simulink model "BD_PAR_SS"  (Simulink 10.3)
settings: Solver=ode1  StartTime=0.0  StopTime=max(cyc_mph(:,1))  FixedStep=1  MaxStep=1  RelTol=1e-3  AbsTol=1e-3
undefined symbols (not defined in the file): acc_elec_eff, acc_elec_pwr, acc_mech_eff, amb_tmp, cs_charge_deplete_bool, cs_electric_decel_spd, cs_electric_launch_spd_hi, cs_electric_launch_spd_lo, cs_hi_soc, cs_lo_soc, cs_off_trq_frac, cyc_avg_time, cyc_cargo_mass, cyc_elevation_init, cyc_filter_bool, cyc_grade, cyc_mph, ess_module_num, ess_on, ess_voc, ex_calc, ex_cat_co_frac, ex_cat_ext_cp, ex_cat_ext_emisv, ex_cat_ext_init_tmp, ex_cat_ext_mass, ex_cat_ext_sarea, ex_cat_hc_frac, ex_cat_i2p_th_cond, ex_cat_i2x_emisv, ex_cat_i2x_th_cond, ex_cat_int_cp, ex_cat_int_init_tmp, ex_cat_int_mass, ex_cat_int_sarea, ex_cat_lim, ex_cat_m2i_th_cond, ex_cat_m2i_tmp, ex_cat_m2p_emisv, ex_cat_mon_cp, ex_cat_mon_init_tmp, ex_cat_mon_mass, ex_cat_mon_sarea, ex_cat_monf_sarea, ex_cat_moni_sarea, ex_cat_nox_frac, ex_cat_p2x_th_cond, ex_cat_pcm_ecp, ex_cat_pcm_mass, ex_cat_pcm_tmp, ex_cat_pipe_cp, ex_cat_pipe_emisv, ex_cat_pipe_init_tmp, ex_cat_pipe_mass, ex_cat_pipe_sarea, ex_cat_pm_frac, ex_cat_tmp_range, ex_gas_cp, ex_manif_cp, ex_manif_emisv ... (+73)
libraries: lib_controls x6, lib_vehicle x3, lib_accessory x2, lib_interactive x1, lib_energy_storage x1, lib_fuel_converter x1
(part 6 of 6)

== system BD_PAR_SS/exhaust sys <ex>/removal efficiencies/removal efficiencies ORNL/NOx_Eff ==
  vol_flow : Inport
  Ex_temp : Inport  Port=2
  HC_Inlet : Inport  Port=3
  NOx_Inlet : Inport  Port=4
  1 : Constant
  >eps : Saturate  UpperLimit=inf  LowerLimit=eps
  Gain : Gain  Gain=2.875  SaturateOnIntegerOverflow=on
  Gain1 : Gain  Gain=.01  SaturateOnIntegerOverflow=on
  HNR : Product  Inputs=*/  SaturateOnIntegerOverflow=on
  HNR^.5 : Math  Operator=sqrt  SaturateOnIntegerOverflow=on
  HNR^2 : Math  Operator=square  SaturateOnIntegerOverflow=on
  HNR^3 : Product  SaturateOnIntegerOverflow=on
  NOx_conv2 : Display
  SV^.5 : Math  Operator=sqrt  SaturateOnIntegerOverflow=on
  SV^2 : Math  Operator=square  SaturateOnIntegerOverflow=on
  SV^3 : Product  SaturateOnIntegerOverflow=on
  Saturation : Saturate  UpperLimit=1.0  LowerLimit=0.0
  Sum : Sum  Inputs=|+++++  SaturateOnIntegerOverflow=on
  Sum1 : Sum  Inputs=|++++  SaturateOnIntegerOverflow=on
  Sum2 : Sum  Inputs=|++++  SaturateOnIntegerOverflow=on
  Sum3 : Sum  Inputs=|+++  SaturateOnIntegerOverflow=on
  TR : Product  Inputs=*/  SaturateOnIntegerOverflow=on
  T^-.5 : Math  Operator=sqrt  SaturateOnIntegerOverflow=on
  T^-2 : Math  Operator=square  SaturateOnIntegerOverflow=on
  T^-3 : Product  SaturateOnIntegerOverflow=on
  b0 : Constant  Value=-1.2477959e2
  b1 : Gain  Gain=-6.671239E-4  SaturateOnIntegerOverflow=on
  b10 : Gain  Gain=-1.7874225E1  SaturateOnIntegerOverflow=on
  b11 : Gain  Gain=-2.0607707  SaturateOnIntegerOverflow=on
  b12 : Gain  Gain=1.3883777E-1  SaturateOnIntegerOverflow=on
  b13 : Gain  SaturateOnIntegerOverflow=on
  b2 : Gain  Gain=8.308073E-2  SaturateOnIntegerOverflow=on
  b3 : Gain  Gain=7.9852675E-9  SaturateOnIntegerOverflow=on
  b4 : Gain  Gain=-3.7023358E-14  SaturateOnIntegerOverflow=on
  b5 : Gain  Gain=-5.4929168E4  SaturateOnIntegerOverflow=on
  b6 : Gain  Gain=4.9229015e3  SaturateOnIntegerOverflow=on
  b7 : Gain  Gain=2.959987e6  SaturateOnIntegerOverflow=on
  b8 : Gain  Gain=-1.022441e8  SaturateOnIntegerOverflow=on
  b9 : Gain  Gain=1.3710201E1  SaturateOnIntegerOverflow=on
  NOx_eff : Outport
  wires:
  >eps/1 -> HNR/2
  NOx_Inlet/1 -> >eps/1
  Saturation/1 -> NOx_eff/1, NOx_conv2/1
  Ex_temp/1 -> TR/2
  HC_Inlet/1 -> HNR/1
  b13/1 -> SV^3/1, b1/1, SV^2/1, SV^.5/1
  Gain1/1 -> Saturation/1
  Sum3/1 -> Gain1/1
  Gain/1 -> HNR^2/1, HNR^3/2, b9/1, HNR^.5/1
  HNR/1 -> Gain/1
  Sum/1 -> Sum3/1
  Sum1/1 -> Sum3/2
  Sum2/1 -> Sum3/3
  b12/1 -> Sum2/4
  b11/1 -> Sum2/3
  b10/1 -> Sum2/2
  b9/1 -> Sum2/1
  HNR^.5/1 -> b10/1
  HNR^2/1 -> b11/1, HNR^3/1
  HNR^3/1 -> b12/1
  b8/1 -> Sum1/4
  b7/1 -> Sum1/3
  b6/1 -> Sum1/2
  b5/1 -> Sum1/1
  T^-.5/1 -> b6/1
  T^-2/1 -> b7/1, T^-3/1
  T^-3/1 -> b8/1
  TR/1 -> b5/1, T^-3/2, T^-2/1, T^-.5/1
  1/1 -> TR/1
  b3/1 -> Sum/5
  b4/1 -> Sum/4
  b1/1 -> Sum/3
  b2/1 -> Sum/2
  b0/1 -> Sum/1
  SV^.5/1 -> b2/1
  SV^2/1 -> b3/1, SV^3/2
  SV^3/1 -> b4/1
  vol_flow/1 -> b13/1

== system BD_PAR_SS/fuel converter  <fc>/engine speed estimator/no-lag Reset Integrator/dt ==
  Clock : Clock
  Memory1 : Memory  InitialCondition=-0.1
  Sum1 : Sum  Inputs=+-  InputSameDT=on  SaturateOnIntegerOverflow=on  OutDataTypeStr=Inherit: Same as first input
  out_1 : Outport  InitialOutput=0
  wires:
  Sum1/1 -> out_1/1
  Memory1/1 -> Sum1/2
  Clock/1 -> Memory1/1, Sum1/1

== system BD_PAR_SS/fuel converter  <fc>/engine torque/effect of inertia (Nm)/Block NOTES ==
  note: Torque required to accelerate the engine inertia is taken from the engine
      | acceleration, and is assumed to be no less than zero if the trace was missed
      | at all on the previous time step.
      |
      | The torque required to accelerate the engine's inertia is never assumed to
      | be more than the product of the engine's maximum torque and the engine's
      | contribution to the total vehicle inertia.

== system BD_PAR_SS/fuel converter  <fc>/engine torque/effect of inertia (Nm)/engine inertia as a function of total vehicle inertia (generous approximation) ==
  Product : Product  Inputs=*/  InputSameDT=on  RndMeth=Zero  SaturateOnIntegerOverflow=on  OutDataTypeStr=Inherit: Same as first input
  Sum : Sum  Inputs=++|  InputSameDT=on  SaturateOnIntegerOverflow=on  OutDataTypeStr=Inherit: Same as first input
  engine inertia as a fraction of total vehicle inertia  (generous approximation)--denomenator : Fcn  Expr=fc_inertia*(u*fd_ratio/wh_radius)^2
  engine inertia as a fraction of total vehicle inertia  (generous approximation)--numerator : Fcn  Expr=fc_inertia*(u*fd_ratio/wh_radius)^2
  veh mass calc : Subsystem
  Out1 : Outport
  wires:
  [gear_ratio] -> engine inertia as a fraction of total vehicle inertia  (generous approximation)--numerator/1, engine inertia as a fraction of total vehicle inertia  (generous approximation)--denomenator/1
  veh mass calc/1(Out1) -> Sum/1
  engine inertia as a fraction of total vehicle inertia  (generous approximation)--denomenator/1 -> Sum/2
  engine inertia as a fraction of total vehicle inertia  (generous approximation)--numerator/1 -> Product/1
  Sum/1 -> Product/2
  Product/1 -> Out1/1

== system BD_PAR_SS/gearbox <gb>/Pout/Pin, neglecting inertia/make division bombproof/Block NOTES ==
  note: this block added 10 July 2001 by mpo:
      | originally a -eps was added to the denominator by default.
      | However, cases were ecountered where Tin-Tineratia was equal to -eps causing
      | the denominator to be zero. This added checking is more rhobust

== system BD_PAR_SS/mechanical accessory loads <acc>/Mechanical Accessory Loads v2 <acc>/Accessory SDO/mechanical power logging ==
  In1 : Inport
  Gain : Gain  Gain=acc_mech_eff  SaturateOnIntegerOverflow=on  OutDataTypeStr=Inherit: Same as input  ParamDataTypeStr=Inherit: Same as input
  To Workspace6 : ToWorkspace  VariableName=acc_mech_pwr_in_a  SampleTime=-1
  To Workspace8 : ToWorkspace  VariableName=acc_mech_pwr_out_a  SampleTime=-1
  wires:
  Gain/1 -> To Workspace8/1
  In1/1 -> Gain/1, To Workspace6/1

== system BD_PAR_SS/mechanical accessory loads <acc>/Mechanical Accessory Loads v2 <acc>/backward model/mechanical accessories (Nm) ==
  w_APU : Inport
  Mechanical Accessories: Const Mech Var Elect : lib_accessory/Mechanical Accessories: Const Mech Var Elect  SystemSampleTime=-1  VariantActivationTime=update diagram  Latency=0  AutoFrameSizeCalculation=off
  T_acc : Outport
  P_mech_acc : Outport  Port=2
  probes : Outport  Port=3
  wires:
  w_APU/1 -> Mechanical Accessories: Const Mech Var Elect/1
  Mechanical Accessories: Const Mech Var Elect/1 -> T_acc/1
  Mechanical Accessories: Const Mech Var Elect/2 -> P_mech_acc/1
  Mechanical Accessories: Const Mech Var Elect/3 -> probes/1

== system BD_PAR_SS/motor/ controller <mc> par/effect of inertia (Nm)/motor inertia as a function of total vehicle inertia (generous approximation)/veh mass calc ==
  Constant : Constant  Value=veh_mass
  Sum : Sum  Inputs=|++  SaturateOnIntegerOverflow=on
  Out1 : Outport
  wires:
  Sum/1 -> Out1/1
  Constant/1 -> Sum/2
  [veh_cargo_mass] -> Sum/1

== system BD_PAR_SS/vehicle <veh>/record achieved force outputs/force req'd to accelerate (N)1/current veh mass ==
  Constant3 : Constant  Value=veh_mass
  Sum1 : Sum  Inputs=|++  SaturateOnIntegerOverflow=on
  Out1 : Outport
  wires:
  Constant3/1 -> Sum1/1
  [veh_cargo_mass] -> Sum1/2
  Sum1/1 -> Out1/1

== system BD_PAR_SS/vehicle <veh>/record achieved force outputs/force req'd to ascend (N)1/current veh mass ==
  Constant3 : Constant  Value=veh_mass
  Sum1 : Sum  Inputs=|++  SaturateOnIntegerOverflow=on
  Out1 : Outport
  wires:
  Constant3/1 -> Sum1/1
  [veh_cargo_mass] -> Sum1/2
  Sum1/1 -> Out1/1

== system BD_PAR_SS/<vc> par/pre-TX parallel gearbox control/shifting1/time since last shift/just shifted ==
  in_1 : Inport
  Memory : Memory  InitialCondition=1
  Relational Operator : RelationalOperator  Operator=~=  RndMeth=Nearest  InputSameDT=on
  out_1 : Outport  InitialOutput=0
  wires:
  in_1/1 -> Memory/1, Relational Operator/2
  Memory/1 -> Relational Operator/1
  Relational Operator/1 -> out_1/1

== system BD_PAR_SS/<vc> par/pre-TX parallel gearbox control/shifting1/time since last shift/timer ==
  trigger : Inport
  Constant : Constant
  Constant1 : Constant  Value=0
  Constant2 : Constant  Value=0
  Switch : Switch  Threshold=eps  SaturateOnIntegerOverflow=on  InputSameDT=on
  no-lag Reset Integrator : Subsystem  mask(No-lag Reset Integrator){initval=15}
      mask prompts: initval "Initial Value"
      mask help: No-lag Reset Integrator
      mask Help: Integrates first input using Euler technique.\nAt the time step that input 2 <> zero,\noutput is reset to input 3.
      mask Display: disp('1/s\nw/ reset\nno lag')
  time : Outport  InitialOutput=0
  wires:
  no-lag Reset Integrator/1(out_1) -> Switch/3
  Constant1/1 -> no-lag Reset Integrator/3(in_3)
  Constant/1 -> no-lag Reset Integrator/1(in_1)
  Constant2/1 -> Switch/1
  trigger/1 -> no-lag Reset Integrator/2(in_2), Switch/2
  Switch/1 -> time/1

== system BD_PAR_SS/fuel converter  <fc>/engine torque/effect of inertia (Nm)/engine inertia as a function of total vehicle inertia (generous approximation)/veh mass calc ==
  Constant : Constant  Value=veh_mass
  Sum : Sum  Inputs=|++  InputSameDT=on  SaturateOnIntegerOverflow=on  OutDataTypeStr=Inherit: Same as first input
  Out1 : Outport
  wires:
  Sum/1 -> Out1/1
  Constant/1 -> Sum/2
  [veh_cargo_mass] -> Sum/1

== system BD_PAR_SS/<vc> par/pre-TX parallel gearbox control/shifting1/time since last shift/timer/no-lag Reset Integrator ==
  in_1 : Inport
  in_2 : Inport  Port=2
  in_3 : Inport  Port=3
  Constant : Constant  Value=0
  Memory : Memory  InitialCondition=initval
  Product : Product  InputSameDT=on  RndMeth=Zero  SaturateOnIntegerOverflow=on  OutDataTypeStr=Inherit: Same as first input
  Sum : Sum  InputSameDT=on  SaturateOnIntegerOverflow=on  OutDataTypeStr=Inherit: Same as first input
  Switch : Switch  Threshold=eps  SaturateOnIntegerOverflow=on  InputSameDT=on
  dt : Subsystem
  in_2==0 : RelationalOperator  Operator===  RndMeth=Nearest  InputSameDT=on
  out_1 : Outport  InitialOutput=0
  wires:
  Constant/1 -> in_2==0/2
  in_2==0/1 -> Switch/2
  Switch/1 -> Memory/1, out_1/1
  Sum/1 -> Switch/1
  Memory/1 -> Sum/1
  Product/1 -> Sum/2
  dt/1(out_1) -> Product/1
  in_1/1 -> Product/2
  in_2/1 -> in_2==0/1
  in_3/1 -> Switch/3

== system BD_PAR_SS/<vc> par/pre-TX parallel gearbox control/shifting1/time since last shift/timer/no-lag Reset Integrator/dt ==
  Clock : Clock
  Memory1 : Memory  InitialCondition=-1
  Sum1 : Sum  Inputs=+-  InputSameDT=on  SaturateOnIntegerOverflow=on  OutDataTypeStr=Inherit: Same as first input
  out_1 : Outport  InitialOutput=0
  wires:
  Sum1/1 -> out_1/1
  Memory1/1 -> Sum1/2
  Clock/1 -> Memory1/1, Sum1/1
